simulink model "ThreeTank_Control2017a"  (R2017a)
settings: Solver=VariableStepAuto  StartTime=0.0  StopTime=58020  RelTol=1e-3
undefined symbols (not defined in the file or in its folder): Kd_1, Kd_2, Ki_1, Ki_2, Kp_1, Kp_2
libraries: simulink x2
settings Model: Creator=xu_pe  LastModifiedBy=124
settings DataIOCC: ReturnWorkspaceOutputs=on
settings DebuggingCC: SFMachineParentedDataDiag=error
settings SFSimCC: SimUseLocalCustomCode=on
settings RTWCC: RTWUseLocalCustomCode=on

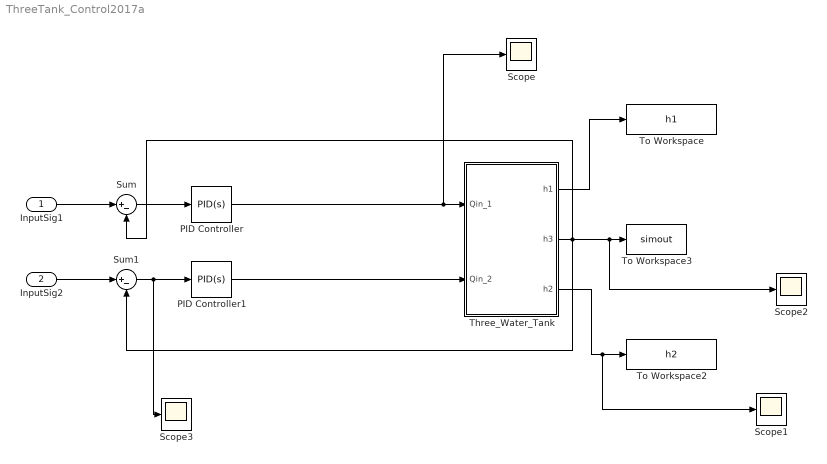
== system ThreeTank_Control2017a ==
  InputSig1 : Inport
  InputSig2 : Inport  Port=2
  PID Controller : simulink/Continuous/PID Controller  Controller=PID  TimeDomain=Continuous-time  SampleTime=-1  IntegratorMethod=Forward Euler  FilterMethod=Forward Euler  Form=Parallel  UseFilter=on  ControllerParametersSource=internal  P=Kp_1  I=Ki_1  D=Kd_1  N=100  InitialConditionSource=internal  InitialConditionForIntegrator=0  InitialConditionForFilter=0  ExternalReset=none  LimitOutput=off  UpperSaturationLimit=inf  LowerSaturationLimit=-inf  LinearizeAsGain=on  AntiWindupMode=none  Kb=1  TrackingMode=off  Kt=1  PParamMin=[]  PParamMax=[]  IParamMin=[]  IParamMax=[]  DParamMin=[]  DParamMax=[]  NParamMin=[]  NParamMax=[]  KbParamMin=[]  KbParamMax=[]  KtParamMin=[]  KtParamMax=[]  POutMin=[]  POutMax=[]  IOutMin=[]  IOutMax=[]  DOutMin=[]  DOutMax=[]  NOutMin=[]  NOutMax=[]  KbOutMin=[]  KbOutMax=[]  KtOutMin=[]  KtOutMax=[]  IntegratorOutMin=[]  IntegratorOutMax=[]  FilterOutMin=[]  FilterOutMax=[]  SumOutMin=[]  SumOutMax=[]  SumI1OutMin=[]  SumI1OutMax=[]  SumI2OutMin=[]  SumI2OutMax=[]  SumI3OutMin=[]  SumI3OutMax=[]  SumDOutMin=[]  SumDOutMax=[]  SaturationOutMin=[]  SaturationOutMax=[]  IntegratorContinuousStateAttributes=''  IntegratorStateMustResolveToSignalObject=off  IntegratorRTWStateStorageClass=Auto  FilterContinuousStateAttributes=''  FilterStateMustResolveToSignalObject=off  FilterRTWStateStorageClass=Auto  DifferentiatorICPrevScaledInput=0  DifferentiatorOutMin=[]  DifferentiatorOutMax=[]  InitialConditionSetting=State (most efficient)
  PID Controller1 : simulink/Continuous/PID Controller  Controller=PID  TimeDomain=Continuous-time  SampleTime=-1  IntegratorMethod=Forward Euler  FilterMethod=Forward Euler  Form=Parallel  UseFilter=on  ControllerParametersSource=internal  P=Kp_2  I=Ki_2  D=Kd_2  N=100  InitialConditionSource=internal  InitialConditionForIntegrator=0  InitialConditionForFilter=0  ExternalReset=none  LimitOutput=off  UpperSaturationLimit=inf  LowerSaturationLimit=-inf  LinearizeAsGain=on  AntiWindupMode=none  Kb=1  TrackingMode=off  Kt=1  PParamMin=[]  PParamMax=[]  IParamMin=[]  IParamMax=[]  DParamMin=[]  DParamMax=[]  NParamMin=[]  NParamMax=[]  KbParamMin=[]  KbParamMax=[]  KtParamMin=[]  KtParamMax=[]  POutMin=[]  POutMax=[]  IOutMin=[]  IOutMax=[]  DOutMin=[]  DOutMax=[]  NOutMin=[]  NOutMax=[]  KbOutMin=[]  KbOutMax=[]  KtOutMin=[]  KtOutMax=[]  IntegratorOutMin=[]  IntegratorOutMax=[]  FilterOutMin=[]  FilterOutMax=[]  SumOutMin=[]  SumOutMax=[]  SumI1OutMin=[]  SumI1OutMax=[]  SumI2OutMin=[]  SumI2OutMax=[]  SumI3OutMin=[]  SumI3OutMax=[]  SumDOutMin=[]  SumDOutMax=[]  SaturationOutMin=[]  SaturationOutMax=[]  IntegratorContinuousStateAttributes=''  IntegratorStateMustResolveToSignalObject=off  IntegratorRTWStateStorageClass=Auto  FilterContinuousStateAttributes=''  FilterStateMustResolveToSignalObject=off  FilterRTWStateStorageClass=Auto  DifferentiatorICPrevScaledInput=0  DifferentiatorOutMin=[]  DifferentiatorOutMax=[]  InitialConditionSetting=State (most efficient)
  Scope{,1..3} (4 alike) : Scope
  Sum : Sum  Inputs=|+-
  Sum1 : Sum  Inputs=|+-
  Three_Water_Tank : Subsystem
  To Workspace : ToWorkspace  VariableName=h1  SaveFormat=Timeseries  SampleTime=-1
  To Workspace2 : ToWorkspace  VariableName=h2  SaveFormat=Timeseries  SampleTime=-1
  To Workspace3 : ToWorkspace  VariableName=simout  SaveFormat=Timeseries  SampleTime=-1
  wires:
  Sum/1 -> PID Controller/1
  Three_Water_Tank/1(h1) -> To Workspace/1
  Three_Water_Tank/2(h3) -> Sum/2, Sum1/2, To Workspace3/1, Scope2/1
  Three_Water_Tank/3(h2) -> Scope1/1, To Workspace2/1
  PID Controller/1 -> Scope/1, Three_Water_Tank/1(Qin_1)
  PID Controller1/1 -> Three_Water_Tank/2(Qin_2)
  Sum1/1 -> Scope3/1, PID Controller1/1
  InputSig1/1 -> Sum/1
  InputSig2/1 -> Sum1/1

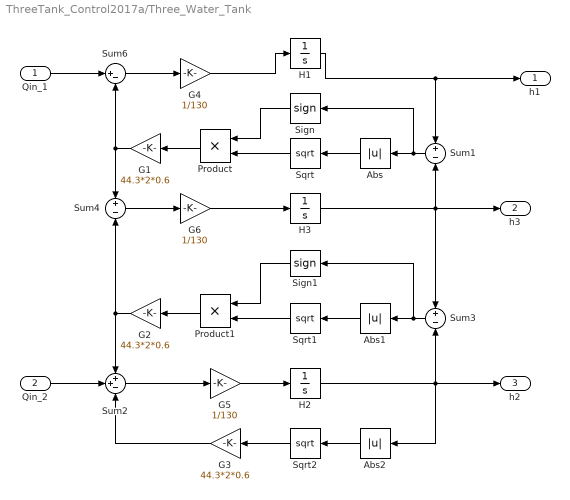
== system ThreeTank_Control2017a/Three_Water_Tank ==
  Qin_1 : Inport  PortDimensions=1  SampleTime=1
  Qin_2 : Inport  Port=2  PortDimensions=1  SampleTime=1
  Abs : Abs  ZeroCross=off
  Abs1 : Abs  ZeroCross=off
  Abs2 : Abs  ZeroCross=off
  G1 : Gain  Gain=44.3*2*0.6
  G2 : Gain  Gain=44.3*2*0.6
  G3 : Gain  Gain=44.3*2*0.6
  G4 : Gain  Gain=1/130
  G5 : Gain  Gain=1/130
  G6 : Gain  Gain=1/130
  H1 : Integrator  InitialCondition=0.0001
  H2 : Integrator  InitialCondition=0.001
  H3 : Integrator  InitialCondition=0.0001
  Product : Product
  Product1 : Product
  Sign : Signum  ZeroCross=off
  Sign1 : Signum  ZeroCross=off
  Sqrt : Sqrt  SaturateOnIntegerOverflow=on
  Sqrt1 : Sqrt  SaturateOnIntegerOverflow=on
  Sqrt2 : Sqrt  SaturateOnIntegerOverflow=on
  Sum1 : Sum  Inputs=+-
  Sum2 : Sum  Inputs=++-
  Sum3 : Sum  Inputs=+-
  Sum4 : Sum  Inputs=+-
  Sum6 : Sum  Inputs=|+-
  h1 : Outport  PortDimensions=1  SampleTime=1
  h3 : Outport  Port=2  PortDimensions=1  SampleTime=1
  h2 : Outport  Port=3  PortDimensions=1  SampleTime=1
  wires:
  Sqrt/1 -> Product/2
  Sqrt1/1 -> Product1/2
  Sum1/1 -> Sign/1, Abs/1
  Sign/1 -> Product/1
  Sum2/1 -> G5/1
  Abs1/1 -> Sqrt1/1
  Sum3/1 -> Sign1/1, Abs1/1
  Sign1/1 -> Product1/1
  Qin_1/1 -> Sum6/1
  G4/1 -> H1/1
  G2/1 -> Sum2/1, Sum4/2
  G6/1 -> H3/1
  Product1/1 -> G2/1
  H1/1 -> h1/1, Sum1/1
  G1/1 -> Sum6/2, Sum4/1
  Sum4/1 -> G6/1
  H3/1 -> Sum3/1, h3/1, Sum1/2
  G3/1 -> Sum2/3
  Sum6/1 -> G4/1
  Sqrt2/1 -> G3/1
  H2/1 -> Abs2/1, h2/1, Sum3/2
  G5/1 -> H2/1
  Abs/1 -> Sqrt/1
  Product/1 -> G1/1
  Qin_2/1 -> Sum2/2
  Abs2/1 -> Sqrt2/1
